simulink model "Simple_3_Model"  (R2022b)
settings: Solver=FixedStepAuto  StartTime=0.0  StopTime=1000  FixedStep=.05  RelTol=1e-3
undefined symbols (not defined in the file or in its folder): importedData
libraries: matrix_library x9
(part 2 of 2)

== matlab function Simple_3_Model/Physics Sim/Wrench Calculation/Linear Drag/Seperate to World Compents ==
  data: x output; robotFrameVelocity input; y output; z output
function [x, y, z] = fcn(robotFrameVelocity)

x = robotFrameVelocity(1, 1);
y = robotFrameVelocity(2, 1);
z = robotFrameVelocity(3, 1);

== matlab function Simple_3_Model/Physics Sim/Wrench Calculation/Angular Drag/Concatenate Drag ==
  data: roll input; velocityVector output; pitch input; yaw input
function velocityVector = fcn(roll,pitch,yaw)

velocityVector = [roll; pitch; yaw];

== matlab function Simple_3_Model/Physics Sim/Wrench Calculation/Angular Drag/Concatenate Velocity ==
  data: row input; column output
function column = fcn(row)

column = [row(1); row(2); row(3)];

== matlab function Simple_3_Model/Physics Sim/Wrench Calculation/Angular Drag/Create Rotation Matrix ==
  data: inverse output; angularPosition input; rotation output
function [inverse, rotation] = fcn(angularPosition)

rotation = eul2rotm([deg2rad(angularPosition(1)), deg2rad(angularPosition(2)), deg2rad(angularPosition(3))]);
inverse = transpose(rotation);

== matlab function Simple_3_Model/Physics Sim/Wrench Calculation/Angular Drag/Seperate to Components ==
  data: roll output; pitch output; yaw output; robotFrameVelocity input
function [roll, pitch, yaw] = fcn(robotFrameVelocity)

roll = robotFrameVelocity(1, 1);
pitch = robotFrameVelocity(2, 1);
yaw = robotFrameVelocity(3, 1);

== matlab function Simple_3_Model/Physics Sim/Wrench Calculation/Angular Drag/Seperate to World Compents ==
  data: roll output; robotFrameVelocity input; pitch output; yaw output
function [roll, pitch, yaw] = fcn(robotFrameVelocity)

roll = robotFrameVelocity(1, 1);
pitch = robotFrameVelocity(2, 1);
yaw = robotFrameVelocity(3, 1);

== matlab function Simple_3_Model/Physics Sim/Wrench Calculation/Thruster Forces and Moments/VUS Thruster/Euler to Unit ==
  data: euler input; direction output
function direction = fcn(euler)

directionCol = eul2rotm(euler, "XYZ") * [1; 0; 0];
direction = [directionCol(1,1), directionCol(2,1), directionCol(3,1)];
